simulink model "Microgrid"  (R2024a)
settings: Solver=VariableStepAuto  StartTime=0.0  StopTime=5  RelTol=1e-3
(part 2 of 2)

== matlab function Microgrid/media ==
  data: u input; y output
function y = media(u)

y = mean(u);
